simulink model "be_step1"  (R2022b)
settings: Solver=VariableStepAuto  StartTime=0.0  StopTime=25  RelTol=1e-3
settings Model: Creator=queinnec  LastModifiedBy=Akash
settings SolverCC: AlgebraicLoopSolver=TrustRegion
settings DataIOCC: ReturnWorkspaceOutputs=off
settings DebuggingCC: UnconnectedInputMsg=warning  UnconnectedOutputMsg=warning  UnconnectedLineMsg=warning  SFMachineParentedDataDiag=warning  ArithmeticOperatorsInVariantConditions=warning
settings ModelReferenceCC: EnableRefExpFcnMdlSchedulingChecks=on
settings SFSimCC: SimUseLocalCustomCode=off  CustomCodeUndefinedFunction=UseInterfaceOnly
settings RTWCC: RTWUseLocalCustomCode=off

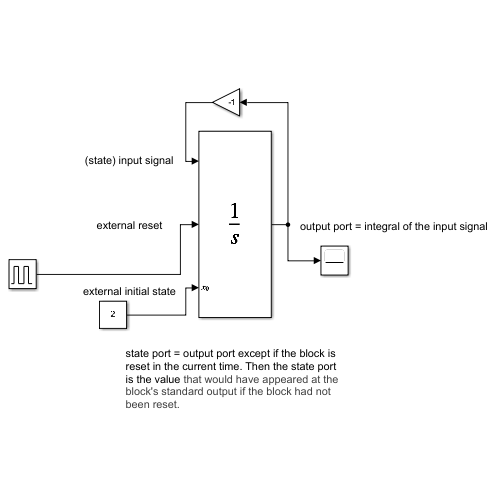
[thumbnail: Simulink's stored preview of the top-level diagram]
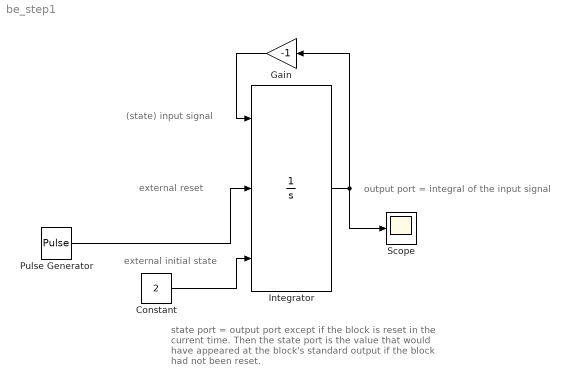
== system be_step1 ==
  note: external initial state
  note: (state) input signal
  note: output port = integral of the input signal
  note: state port = output port except if the block is reset in the current time. Then the state port is the value that would have appeared at the block's standard output if the block had not been reset.
  note: external reset
  Constant : Constant  Value=2
  Gain : Gain  Gain=-1
  Integrator : Integrator  ExternalReset=level hold  InitialConditionSource=external  ZeroCross=off
  Pulse Generator : DiscretePulseGenerator  PulseType=Time based  Period=5  PulseWidth=0.0001
  Scope : Scope
  wires:
  Constant/1 -> Integrator/3
  Pulse Generator/1 -> Integrator/2
  Integrator/1 -> Scope/1, Gain/1
  Gain/1 -> Integrator/1
